simulink model "xpos_control"  (R2015a)
settings: Solver=ode45  StartTime=0.0  StopTime=50  RelTol=1e-3
undefined symbols (not defined in the file or in its folder): Grx, rrx
libraries: cstblocks x5, simulink x1
settings Model: Creator=morten  LastModifiedBy=morten

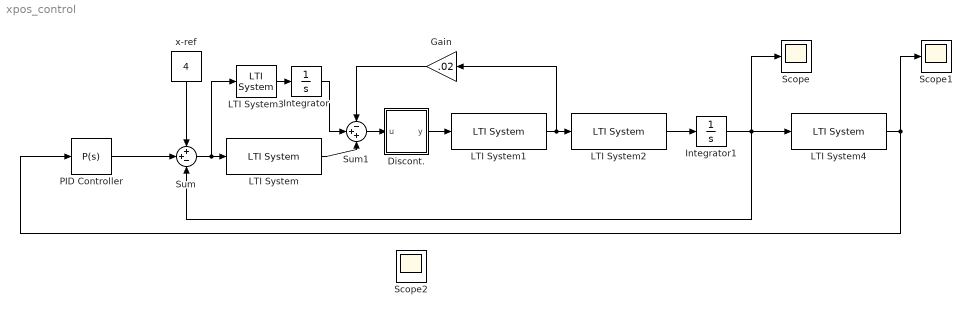
== system xpos_control ==
  Discont. : MATLAB Function  TreatAsAtomicUnit=on
  Gain : Gain  Gain=.02
  Integrator : Integrator  LimitOutput=on  UpperSaturationLimit=2.500  LowerSaturationLimit=-2.500
  Integrator1 : Integrator  LowerSaturationLimit=-2.500
  LTI System : cstblocks/LTI System  sys=C1_p  IC=[]
  LTI System1 : cstblocks/LTI System  sys=Mx  IC=[]
  LTI System2 : cstblocks/LTI System  sys=Grx*rrx  IC=[]
  LTI System3 : cstblocks/LTI System  sys=C1_i  IC=[]
  LTI System4 : cstblocks/LTI System  sys=W  IC=[]
  PID Controller : simulink/Continuous/PID Controller  Controller=P  TimeDomain=Continuous-time  SampleTime=-1  IntegratorMethod=Forward Euler  FilterMethod=Forward Euler  Form=Parallel  UseFilter=on  ControllerParametersSource=internal  P=10  I=1  D=.1  N=100  InitialConditionSource=internal  InitialConditionForIntegrator=0  InitialConditionForFilter=0  ExternalReset=none  LimitOutput=off  UpperSaturationLimit=inf  LowerSaturationLimit=-inf  LinearizeAsGain=on  AntiWindupMode=none  Kb=1  TrackingMode=off  Kt=1  PParamMin=[]  PParamMax=[]  IParamMin=[]  IParamMax=[]  DParamMin=[]  DParamMax=[]  NParamMin=[]  NParamMax=[]  KbParamMin=[]  KbParamMax=[]  KtParamMin=[]  KtParamMax=[]  POutMin=[]  POutMax=[]  IOutMin=[]  IOutMax=[]  DOutMin=[]  DOutMax=[]  NOutMin=[]  NOutMax=[]  KbOutMin=[]  KbOutMax=[]  KtOutMin=[]  KtOutMax=[]  IntegratorOutMin=[]  IntegratorOutMax=[]  FilterOutMin=[]  FilterOutMax=[]  SumOutMin=[]  SumOutMax=[]  SumI1OutMin=[]  SumI1OutMax=[]  SumI2OutMin=[]  SumI2OutMax=[]  SumI3OutMin=[]  SumI3OutMax=[]  SumDOutMin=[]  SumDOutMax=[]  SaturationOutMin=[]  SaturationOutMax=[]  IntegratorContinuousStateAttributes=''  IntegratorStateMustResolveToSignalObject=off  IntegratorRTWStateStorageClass=Auto  FilterContinuousStateAttributes=''  FilterStateMustResolveToSignalObject=off  FilterRTWStateStorageClass=Auto  DifferentiatorICPrevScaledInput=0  DifferentiatorOutMin=[]  DifferentiatorOutMax=[]
  Scope : Scope
  Scope1 : Scope
  Scope2 : Scope
      settings: SaveName=ScopeData2
  Sum : Sum  Inputs=++-
  Sum1 : Sum  Inputs=-++
  x-ref : Constant  Value=4
  wires:
  x-ref/1 -> Sum/1
  Sum/1 -> LTI System3/1, LTI System/1
  LTI System/1 -> Sum1/3
  LTI System2/1 -> Integrator1/1
  LTI System3/1 -> Integrator/1
  Integrator/1 -> Sum1/2
  Sum1/1 -> Discont./1(u)
  Integrator1/1 -> Sum/3, LTI System4/1, Scope/1
  LTI System1/1 -> Gain/1, LTI System2/1
  Gain/1 -> Sum1/1
  LTI System4/1 -> PID Controller/1, Scope1/1
  PID Controller/1 -> Sum/2
  Discont./1(y) -> LTI System1/1

== matlab function xpos_control/Discont. ==
  data: u input; y output
function y = dis(u)
    if(u > -4.6 && u < -0.2)
        y = -4.6;
    elseif(u < 4.6 && u > 0.2)
        y = 4.6;
    elseif( u < 0.2 && u > -0.2)
        y = 0;
    elseif(u > 12.5)
        y = 12.5;
    elseif(u < -12.5)
        y = -12.5;
    else
        y = u;
end
